simulink model "h2omnix_heading_coop"  (R2022b)
settings: Solver=ode4  StartTime=0.0  StopTime=inf  FixedStep=0.05  RelTol=1e-3
InitFcn:
  | simulacija
undefined symbols (not defined in the file): nu_max, nu_min, pcKd, pcKp, PD_Fil, PD_Filc, PD_Kd, PD_Kdc, PD_Kp, PD_Kpc, vcKi, vcKic, vcKp, vcKpc, vcKt, vcKtc, wn
libraries: MarineRoboticsLib x6, MarineRoboticsLibEx x2, slpidlib x2, matrix_library x2
settings Model: DataDictionary=ros2lib.sldd  Creator=dnad  LastModifiedBy=Zarko Zecevic

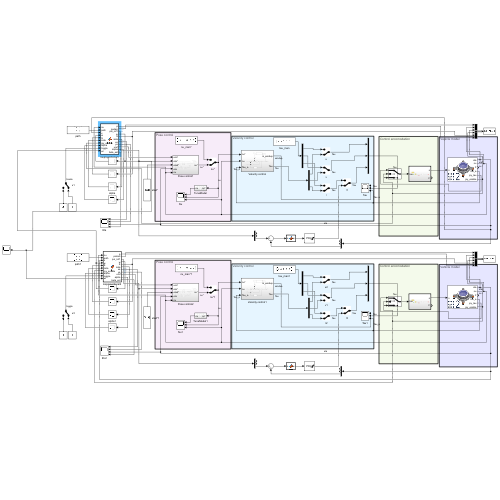
[thumbnail: Simulink's stored preview of the top-level diagram]
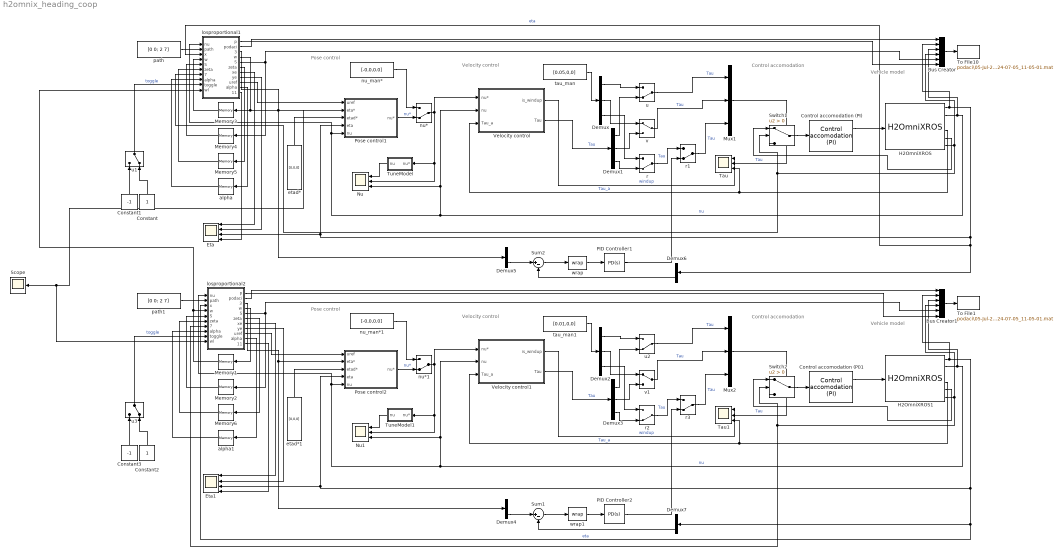
== system h2omnix_heading_coop ==
  note: Control accomodation
  note: Vehicle model
  note: Pose control
  note: Velocity control
  note: Velocity control
  note: Vehicle model
  note: Pose control
  note: Control accomodation
  Bus Creator : BusCreator  Inputs=6
  Bus Creator1 : BusCreator  Inputs=6
  Constant : Constant
  Constant1 : Constant  Value=-1
  Constant2 : Constant
  Constant3 : Constant  Value=-1
  Control accomodation (PI) : MarineRoboticsLibEx/Control accomodation (PI)  SystemSampleTime=-1  VariantActivationTime=update diagram  Latency=0  AutoFrameSizeCalculation=off
  Control accomodation (PI)1 : MarineRoboticsLibEx/Control accomodation (PI)  SystemSampleTime=-1  VariantActivationTime=update diagram  Latency=0  AutoFrameSizeCalculation=off
  Demux{,1..7} (8 alike) : Demux  Outputs=3
  Eta : Scope  NumInputPorts=4
  Eta1 : Scope  NumInputPorts=4
  H2OmniXROS : MarineRoboticsLib/H2OmniXROS  vehicle_name=krk  max_pwm=0.4  pwm_topic=/krk/pwm_out  joy_topic=/krk/joy  odometry_topic=/krk/odometry/filtered
  H2OmniXROS1 : MarineRoboticsLib/H2OmniXROS  vehicle_name=cres  max_pwm=0.4  pwm_topic=/cres/pwm_out  joy_topic=/cres/joy  odometry_topic=/cres/odometry/filtered
  Memory1 : Memory  InitialCondition=1
  Memory2 : Memory  InitialCondition=0.1*eye(3)
  Memory3 : Memory  InitialCondition=1
  Memory4 : Memory  InitialCondition=0.1*eye(3)
  Memory5 : Memory  InitialCondition=[0;0;0]
  Memory6 : Memory  InitialCondition=[0;0;0]
  Mux1 : Mux  Inputs=3
  Mux2 : Mux  Inputs=3
  Nu : Scope  NumInputPorts=3
  Nu1 : Scope  NumInputPorts=3
  PID Controller1 : slpidlib/PID Controller  Controller=PD  Form=Parallel  TimeDomain=Continuous-time  UseExternalTs=off  SampleTime=-1  IntegratorMethod=Forward Euler  FilterMethod=Forward Euler  ControllerParametersSource=internal  P=PD_Kp  I=1  UseKiTs=off  D=PD_Kd  N=PD_Fil  UseFilter=on  TunerSelectOption=Transfer Function Based (PID Tuner App)  InitialConditionSource=internal  InitialConditionForIntegrator=0  InitialConditionForFilter=0  DifferentiatorICPrevScaledInput=0  ExternalReset=none  TrackingMode=off  Kt=1  LimitOutput=on  SatLimitsSource=internal  UpperSaturationLimit=0.8  LowerSaturationLimit=-0.8  LinearizeAsGain=on  AntiWindupMode=none  Kb=1  LimitIntegrator=off  UpperIntegratorSaturationLimit=inf  LowerIntegratorSaturationLimit=-inf  POutMin=[]  POutMax=[]  IOutMin=[]  IOutMax=[]  DOutMin=[]  DOutMax=[]  NOutMin=[]  NOutMax=[]  SumOutMin=[]  SumOutMax=[]  SaturationOutMin=[]  SaturationOutMax=[]  PParamMin=[]  PParamMax=[]  IParamMin=[]  IParamMax=[]  DParamMin=[]  DParamMax=[]  NParamMin=[]  NParamMax=[]  KbParamMin=[]  KbParamMax=[]  KtParamMin=[]  KtParamMax=[]  KbOutMin=[]  KbOutMax=[]  KtOutMin=[]  KtOutMax=[]  IntegratorOutMin=[]  IntegratorOutMax=[]  FilterOutMin=[]  FilterOutMax=[]  SumI1OutMin=[]  SumI1OutMax=[]  SumI2OutMin=[]  SumI2OutMax=[]  SumI3OutMin=[]  SumI3OutMax=[]  SumI4OutMin=[]  SumI4OutMax=[]  SumDOutMin=[]  SumDOutMax=[]  DifferentiatorOutMin=[]  DifferentiatorOutMax=[]  FilterDiffOutCoefMin=[]  FilterDiffOutCoefMax=[]  ReciprocalOutMin=[]  ReciprocalOutMax=[]  SumDenOutMin=[]  SumDenOutMax=[]  SumNumOutMin=[]  SumNumOutMax=[]  DivideOutMin=[]  DivideOutMax=[]  UdiffTsProdOutMin=[]  UdiffTsProdOutMax=[]  NTsProdOutMin=[]  NTsProdOutMax=[]  UintegralTsProdOutMin=[]  UintegralTsProdOutMax=[]  UngainTsProdOutMin=[]  UngainTsProdOutMax=[]  ClampingZeroOutDataTypeStr=Inherit: Inherit via back propagation  ClampingZeroOutMin=[]  ClampingZeroOutMax=[]  FilterDenConstantOutDataTypeStr=Inherit: Inherit via back propagation  FilterDenConstantOutMin=[]  FilterDenConstantOutMax=[]  PCopyOutDataTypeStr=Inherit: Inherit via back propagation  PCopyOutMin=[]  PCopyOutMax=[]  NCopyOutDataTypeStr=Inherit: Inherit via back propagation  NCopyOutMin=[]  NCopyOutMax=[]  IntegratorContinuousStateAttributes=''  IntegratorStateMustResolveToSignalObject=off  IntegratorRTWStateStorageClass=Auto  FilterContinuousStateAttributes=''  FilterStateMustResolveToSignalObject=off  FilterRTWStateStorageClass=Auto  ParallelPVariant=InternalParameters  IdealPVariant=Disabled  IVariant=Disabled  DVariant=InternalParameters  IntegratorVariant=Disabled  SatVariant=Enabled  AWVariant=Disabled  PCopyVariant=Disabled  TRVariant=Disabled  FdbkBlocksVariant=Forward  IdealPFdbkVariant=Disabled  SatFdbkVariant=Disabled  DerivativeFilterVariant=ContFilter  NVariant=InternalParameters  NCopyVariant=Disabled  FilterICVariant=InternalICsFilter  IntegratorICVariant=Disabled  ExternalResetVariant=Disabled  TRSumVariant=Passthrough  SumFdbkVariant=Disabled  SumVariant=Sum_PD  TsampFilterVariant=InternalTs  TsampNgainVariant=Passthrough  TsampIntegralVariant=Disabled_SignalSpec  ExternalSaturationOutDataTypeStr=Inherit: Same as second input
  PID Controller2 : slpidlib/PID Controller  Controller=PD  Form=Parallel  TimeDomain=Continuous-time  UseExternalTs=off  SampleTime=-1  IntegratorMethod=Forward Euler  FilterMethod=Forward Euler  ControllerParametersSource=internal  P=PD_Kpc  I=1  UseKiTs=off  D=PD_Kdc  N=PD_Filc  UseFilter=on  TunerSelectOption=Transfer Function Based (PID Tuner App)  InitialConditionSource=internal  InitialConditionForIntegrator=0  InitialConditionForFilter=0  DifferentiatorICPrevScaledInput=0  ExternalReset=none  TrackingMode=off  Kt=1  LimitOutput=on  SatLimitsSource=internal  UpperSaturationLimit=0.8  LowerSaturationLimit=-0.8  LinearizeAsGain=on  AntiWindupMode=none  Kb=1  LimitIntegrator=off  UpperIntegratorSaturationLimit=inf  LowerIntegratorSaturationLimit=-inf  POutMin=[]  POutMax=[]  IOutMin=[]  IOutMax=[]  DOutMin=[]  DOutMax=[]  NOutMin=[]  NOutMax=[]  SumOutMin=[]  SumOutMax=[]  SaturationOutMin=[]  SaturationOutMax=[]  PParamMin=[]  PParamMax=[]  IParamMin=[]  IParamMax=[]  DParamMin=[]  DParamMax=[]  NParamMin=[]  NParamMax=[]  KbParamMin=[]  KbParamMax=[]  KtParamMin=[]  KtParamMax=[]  KbOutMin=[]  KbOutMax=[]  KtOutMin=[]  KtOutMax=[]  IntegratorOutMin=[]  IntegratorOutMax=[]  FilterOutMin=[]  FilterOutMax=[]  SumI1OutMin=[]  SumI1OutMax=[]  SumI2OutMin=[]  SumI2OutMax=[]  SumI3OutMin=[]  SumI3OutMax=[]  SumI4OutMin=[]  SumI4OutMax=[]  SumDOutMin=[]  SumDOutMax=[]  DifferentiatorOutMin=[]  DifferentiatorOutMax=[]  FilterDiffOutCoefMin=[]  FilterDiffOutCoefMax=[]  ReciprocalOutMin=[]  ReciprocalOutMax=[]  SumDenOutMin=[]  SumDenOutMax=[]  SumNumOutMin=[]  SumNumOutMax=[]  DivideOutMin=[]  DivideOutMax=[]  UdiffTsProdOutMin=[]  UdiffTsProdOutMax=[]  NTsProdOutMin=[]  NTsProdOutMax=[]  UintegralTsProdOutMin=[]  UintegralTsProdOutMax=[]  UngainTsProdOutMin=[]  UngainTsProdOutMax=[]  ClampingZeroOutDataTypeStr=Inherit: Inherit via back propagation  ClampingZeroOutMin=[]  ClampingZeroOutMax=[]  FilterDenConstantOutDataTypeStr=Inherit: Inherit via back propagation  FilterDenConstantOutMin=[]  FilterDenConstantOutMax=[]  PCopyOutDataTypeStr=Inherit: Inherit via back propagation  PCopyOutMin=[]  PCopyOutMax=[]  NCopyOutDataTypeStr=Inherit: Inherit via back propagation  NCopyOutMin=[]  NCopyOutMax=[]  IntegratorContinuousStateAttributes=''  IntegratorStateMustResolveToSignalObject=off  IntegratorRTWStateStorageClass=Auto  FilterContinuousStateAttributes=''  FilterStateMustResolveToSignalObject=off  FilterRTWStateStorageClass=Auto  ParallelPVariant=InternalParameters  IdealPVariant=Disabled  IVariant=Disabled  DVariant=InternalParameters  IntegratorVariant=Disabled  SatVariant=Enabled  AWVariant=Disabled  PCopyVariant=Disabled  TRVariant=Disabled  FdbkBlocksVariant=Forward  IdealPFdbkVariant=Disabled  SatFdbkVariant=Disabled  DerivativeFilterVariant=ContFilter  NVariant=InternalParameters  NCopyVariant=Disabled  FilterICVariant=InternalICsFilter  IntegratorICVariant=Disabled  ExternalResetVariant=Disabled  TRSumVariant=Passthrough  SumFdbkVariant=Disabled  SumVariant=Sum_PD  TsampFilterVariant=InternalTs  TsampNgainVariant=Passthrough  TsampIntegralVariant=Disabled_SignalSpec  ExternalSaturationOutDataTypeStr=Inherit: Same as second input
  Pose control1 : Subsystem
  Pose control2 : Subsystem
  Scope : Scope
  Sum1 : Sum  Inputs=|+-
  Sum2 : Sum  Inputs=|+-
  Switch1 : Switch  Criteria=u2 > Threshold  SaturateOnIntegerOverflow=off  InputSameDT=off
  Switch2 : Switch  Criteria=u2 > Threshold  SaturateOnIntegerOverflow=off  InputSameDT=off
  Tau : Scope  NumInputPorts=3
  Tau1 : Scope  NumInputPorts=3
  To File1 : ToFile  Filename=podaci\05-Jul-2024\cres_2024-07-05_11-05-01.mat  MatrixName=data  SaveFormat=Timeseries
  To File10 : ToFile  Filename=podaci\05-Jul-2024\krk_2024-07-05_11-05-01.mat  MatrixName=data  SaveFormat=Timeseries
  TuneModel : Subsystem
  TuneModel1 : Subsystem
  Velocity control : Subsystem
  Velocity control1 : Subsystem
  alpha : Memory
  alpha1 : Memory
  etad* : Constant  Value=[0,0,0]
  etad*1 : Constant  Value=[0,0,0]
  losproportional1 : MATLAB Function  TreatAsAtomicUnit=on
  losproportional2 : MATLAB Function  TreatAsAtomicUnit=on
  nu* : ManualSwitch  CurrentSetting=0
  nu*1 : ManualSwitch  CurrentSetting=0
  nu_man* : Constant  Value=[-0,0,0.0]
  nu_man*1 : Constant  Value=[-0,0,0.0]
  path : Constant  Value=[0 0; 2 7]
  path1 : Constant  Value=[0 0; 2 7]
  r{,1..3} (4 alike) : ManualSwitch  CurrentSetting=0
  tau_man : Constant  Value=[0.05,0,0]
  tau_man1 : Constant  Value=[0.01,0,0]
  u{,1..3} (4 alike) : ManualSwitch  CurrentSetting=0
  v : ManualSwitch
  v1 : ManualSwitch
  wrap : MarineRoboticsLib/wrap  SystemSampleTime=-1  VariantActivationTime=update diagram  Latency=0  AutoFrameSizeCalculation=off
      settings: LibrarySourceBlock=|
      | simulink/User-Defined
      | Functions/MATLAB Function
  wrap1 : MarineRoboticsLib/wrap  SystemSampleTime=-1  VariantActivationTime=update diagram  Latency=0  AutoFrameSizeCalculation=off
      settings: LibrarySourceBlock=|
      | simulink/User-Defined
      | Functions/MATLAB Function
  wires:
  Switch1/1 -> Control accomodation (PI)/1
  H2OmniXROS/6 -> losproportional1/7(joy_enable), Switch1/2, Bus Creator/4
  losproportional1/7(xe) -> Eta/1
  Velocity control/1(is_windup) -> Tau/1  "windup"
  etad*/1 -> Pose control1/3(etad*)
  Pose control1/1(nu*) -> nu*/2  "nu*"
  Mux1/1 -> Tau/2, Switch1/3  "Tau"
  TuneModel/1(nu) -> Nu/1
  nu_man*/1 -> nu*/1
  H2OmniXROS/1 -> losproportional1/3(x), Demux6/1, Pose control1/4(eta), Eta/3, Bus Creator/2  "eta"
  H2OmniXROS/2 -> Pose control1/5(nu), losproportional1/1(nu), Velocity control/2(nu), Nu/3, Bus Creator/3  "nu"
  H2OmniXROS/4 -> Velocity control/3(Tau_a), Tau/3  "Tau_a"
  nu*/1 -> Nu/2, TuneModel/1(nu*), Velocity control/1(nu*)
  Velocity control/2(Tau) -> Demux1/1  "Tau"
  Demux/1 -> u/1
  Demux1/1 -> u/2
  Demux/2 -> v/1
  Demux1/2 -> v/2
  Demux/3 -> r/1
  Demux1/3 -> r/2
  v/1 -> Mux1/2  "Tau"
  u/1 -> Mux1/1  "Tau"
  tau_man/1 -> Demux/1
  Control accomodation (PI)/1 -> H2OmniXROS/1
  path/1 -> losproportional1/2(path)
  r/1 -> r1/1  "Tau"
  wrap/1 -> PID Controller1/1
  Sum2/1 -> wrap/1
  PID Controller1/1 -> r1/2
  Demux5/3 -> Sum2/1
  Demux6/3 -> Sum2/2
  r1/1 -> Mux1/3  "Tau"
  H2OmniXROS/5 -> Switch1/1
  Memory3/1 -> losproportional1/4("w ")
  losproportional1/5(S) -> Bus Creator/5, Memory4/1
  Memory4/1 -> losproportional1/5("S ")
  losproportional1/6(zeta) -> Memory5/1
  Memory5/1 -> losproportional1/6("zeta ")
  losproportional1/3(psi_ref1) -> Demux5/1, Pose control1/2(eta*)
  losproportional1/9(uref) -> Pose control1/1(uref)
  losproportional1/2(podaci) -> Bus Creator/1
  Bus Creator/1 -> To File10/1
  losproportional1/10(alpha) -> alpha/1
  alpha/1 -> losproportional1/8("alpha ")
  losproportional1/8(ye) -> Eta/2
  losproportional1/11(beta_est) -> Eta/4
  losproportional1/1(p) -> Bus Creator/6
  u1/1 -> losproportional1/9(toggle)  "toggle"
  Constant/1 -> u1/2
  Constant1/1 -> u1/1
  H2OmniXROS1/1 -> losproportional2/3(x), Demux7/1, Pose control2/4(eta), Eta1/3, Bus Creator1/2  "eta"
  Demux3/1 -> u2/2
  nu*1/1 -> Nu1/2, TuneModel1/1(nu*), Velocity control1/1(nu*)
  TuneModel1/1(nu) -> Nu1/1
  nu_man*1/1 -> nu*1/1
  H2OmniXROS1/4 -> Velocity control1/3(Tau_a), Tau1/3  "Tau_a"
  Mux2/1 -> Tau1/2, Switch2/3  "Tau"
  losproportional2/7(xe) -> Eta1/1
  H2OmniXROS1/2 -> Pose control2/5(nu), losproportional2/1(nu), Velocity control1/2(nu), Nu1/3, Bus Creator1/3  "nu"
  losproportional2/6(zeta) -> Memory6/1
  u3/1 -> losproportional2/9(toggle)  "toggle"
  etad*1/1 -> Pose control2/3(etad*)
  Velocity control1/2(Tau) -> Demux3/1  "Tau"
  losproportional2/2(podaci) -> Bus Creator1/1
  Demux7/3 -> Sum1/2
  losproportional2/11(beta_est) -> Eta1/4
  losproportional2/1(p) -> Bus Creator1/6
  Demux2/2 -> v1/1
  losproportional2/4(w) -> Memory1/1
  alpha1/1 -> losproportional2/8("alpha ")
  Demux2/1 -> u2/1
  Bus Creator1/1 -> To File1/1
  Pose control2/1(nu*) -> nu*1/2  "nu*"
  losproportional2/9(uref) -> Pose control2/1(uref)
  Switch2/1 -> Control accomodation (PI)1/1
  H2OmniXROS1/6 -> losproportional2/7(joy_enable), Switch2/2, Bus Creator1/4
  Memory6/1 -> losproportional2/6("zeta ")
  losproportional2/10(alpha) -> alpha1/1
  Memory2/1 -> losproportional2/5("S ")
  losproportional2/5(S) -> Bus Creator1/5, Memory2/1
  H2OmniXROS1/5 -> Switch2/1
  tau_man1/1 -> Demux2/1
  Sum1/1 -> wrap1/1
  Demux3/3 -> r2/2
  wrap1/1 -> PID Controller2/1
  r3/1 -> Mux2/3  "Tau"
  Demux3/2 -> v1/2
  Demux2/3 -> r2/1
  path1/1 -> losproportional2/2(path)
  Velocity control1/1(is_windup) -> Tau1/1  "windup"
  r2/1 -> r3/1  "Tau"
  Demux4/3 -> Sum1/1
  v1/1 -> Mux2/2  "Tau"
  u2/1 -> Mux2/1  "Tau"
  Constant3/1 -> u3/1
  PID Controller2/1 -> r3/2
  losproportional2/8(ye) -> Eta1/2
  Control accomodation (PI)1/1 -> H2OmniXROS1/1
  Constant2/1 -> u3/2
  losproportional2/3(psi_ref1) -> Demux4/1, Pose control2/2(eta*)
  Memory1/1 -> losproportional1/10(wl), losproportional2/4("w ")
  losproportional1/4(w) -> losproportional2/10(wl), Scope/1, Memory3/1

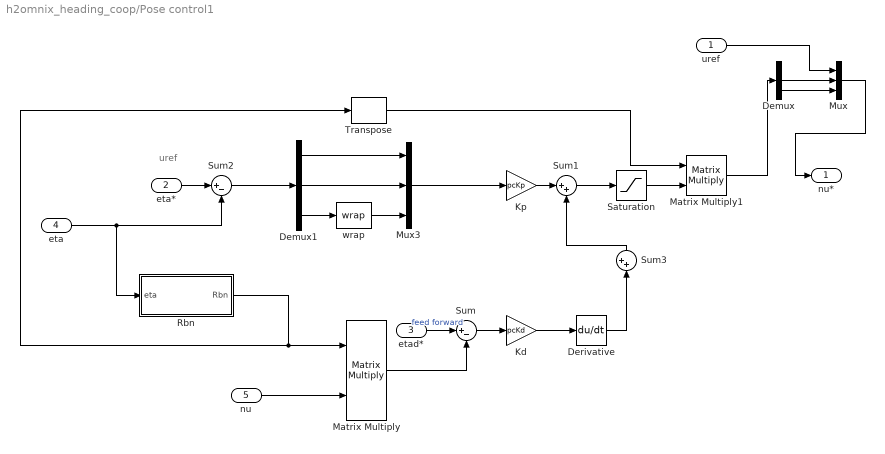
== system h2omnix_heading_coop/Pose control1 ==
  note: uref
  uref : Inport
  eta* : Inport  Port=2
  etad* : Inport  Port=3
  eta : Inport  Port=4
  nu : Inport  Port=5
  Demux : Demux  Outputs=3
  Demux1 : Demux  Outputs=3
  Derivative : Derivative
  Kd : Gain  Gain=pcKd
  Kp : Gain  Gain=pcKp
  Matrix Multiply : Product  Multiplication=Matrix(*)
  Matrix Multiply1 : Product  Multiplication=Matrix(*)
  Mux : Mux  Inputs=3
  Mux3 : Mux  Inputs=3
  Rbn : MATLAB Function  TreatAsAtomicUnit=on
  Saturation : Saturate  UpperLimit=nu_max  LowerLimit=nu_min
  Sum : Sum  Inputs=|+-
  Sum1 : Sum  Inputs=|++
  Sum2 : Sum  Inputs=|+-
  Sum3 : Sum  Inputs=++|
  Transpose : matrix_library/Transpose
  wrap : MarineRoboticsLib/wrap  SystemSampleTime=-1  VariantActivationTime=update diagram  Latency=0  AutoFrameSizeCalculation=off
      settings: LibrarySourceBlock=|
      | simulink/User-Defined
      | Functions/MATLAB Function
  nu* : Outport
  wires:
  Sum/1 -> Kd/1
  eta/1 -> Rbn/1(eta), Sum2/2
  etad*/1 -> Sum/1  "feed forward"
  Kp/1 -> Sum1/1
  eta*/1 -> Sum2/1
  Sum2/1 -> Demux1/1
  Demux1/1 -> Mux3/1
  Demux1/2 -> Mux3/2
  Demux1/3 -> wrap/1
  wrap/1 -> Mux3/3
  Mux3/1 -> Kp/1
  Sum1/1 -> Saturation/1
  Sum3/1 -> Sum1/2
  Kd/1 -> Derivative/1
  Rbn/1(Rbn) -> Matrix Multiply/1, Transpose/1
  Matrix Multiply1/1 -> Demux/1
  Matrix Multiply/1 -> Sum/2
  Saturation/1 -> Matrix Multiply1/2
  Transpose/1 -> Matrix Multiply1/1
  Derivative/1 -> Sum3/2
  nu/1 -> Matrix Multiply/2
  Demux/3 -> Mux/3
  Demux/2 -> Mux/2
  uref/1 -> Mux/1
  Mux/1 -> nu*/1

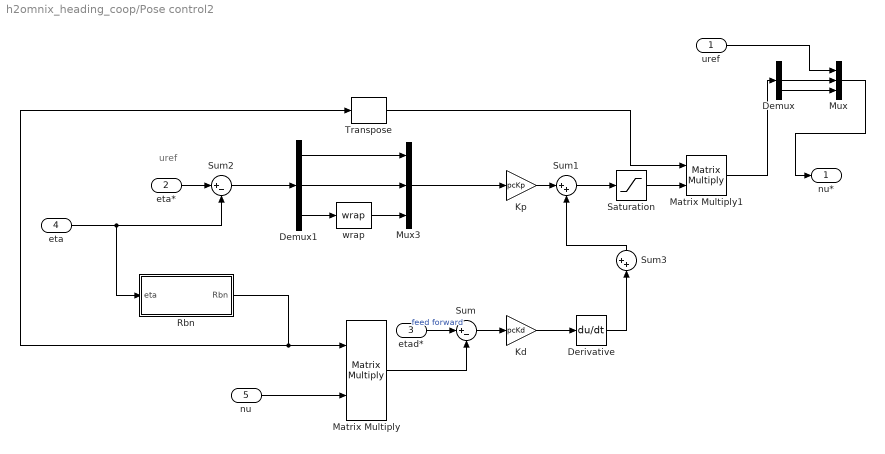
== system h2omnix_heading_coop/Pose control2 ==
  note: uref
  uref : Inport
  eta* : Inport  Port=2
  etad* : Inport  Port=3
  eta : Inport  Port=4
  nu : Inport  Port=5
  Demux : Demux  Outputs=3
  Demux1 : Demux  Outputs=3
  Derivative : Derivative
  Kd : Gain  Gain=pcKd
  Kp : Gain  Gain=pcKp
  Matrix Multiply : Product  Multiplication=Matrix(*)
  Matrix Multiply1 : Product  Multiplication=Matrix(*)
  Mux : Mux  Inputs=3
  Mux3 : Mux  Inputs=3
  Rbn : MATLAB Function  TreatAsAtomicUnit=on
  Saturation : Saturate  UpperLimit=nu_max  LowerLimit=nu_min
  Sum : Sum  Inputs=|+-
  Sum1 : Sum  Inputs=|++
  Sum2 : Sum  Inputs=|+-
  Sum3 : Sum  Inputs=++|
  Transpose : matrix_library/Transpose
  wrap : MarineRoboticsLib/wrap  SystemSampleTime=-1  VariantActivationTime=update diagram  Latency=0  AutoFrameSizeCalculation=off
      settings: LibrarySourceBlock=|
      | simulink/User-Defined
      | Functions/MATLAB Function
  nu* : Outport
  wires:
  Sum/1 -> Kd/1
  eta/1 -> Rbn/1(eta), Sum2/2
  etad*/1 -> Sum/1  "feed forward"
  Kp/1 -> Sum1/1
  eta*/1 -> Sum2/1
  Sum2/1 -> Demux1/1
  Demux1/1 -> Mux3/1
  Demux1/2 -> Mux3/2
  Demux1/3 -> wrap/1
  wrap/1 -> Mux3/3
  Mux3/1 -> Kp/1
  Sum1/1 -> Saturation/1
  Sum3/1 -> Sum1/2
  Kd/1 -> Derivative/1
  Rbn/1(Rbn) -> Matrix Multiply/1, Transpose/1
  Matrix Multiply1/1 -> Demux/1
  Matrix Multiply/1 -> Sum/2
  Saturation/1 -> Matrix Multiply1/2
  Transpose/1 -> Matrix Multiply1/1
  Derivative/1 -> Sum3/2
  nu/1 -> Matrix Multiply/2
  Demux/3 -> Mux/3
  Demux/2 -> Mux/2
  uref/1 -> Mux/1
  Mux/1 -> nu*/1

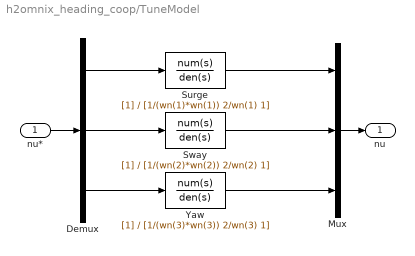
== system h2omnix_heading_coop/TuneModel ==
  nu* : Inport
  Demux : Demux  Outputs=3
  Mux : Mux  Inputs=3
  Surge : TransferFcn  Denominator=[1/(wn(1)*wn(1)) 2/wn(1) 1]
  Sway : TransferFcn  Denominator=[1/(wn(2)*wn(2)) 2/wn(2) 1]
  Yaw : TransferFcn  Denominator=[1/(wn(3)*wn(3)) 2/wn(3) 1]
  nu : Outport
  wires:
  nu*/1 -> Demux/1
  Demux/1 -> Surge/1
  Surge/1 -> Mux/1
  Mux/1 -> nu/1
  Sway/1 -> Mux/2
  Demux/2 -> Sway/1
  Demux/3 -> Yaw/1
  Yaw/1 -> Mux/3

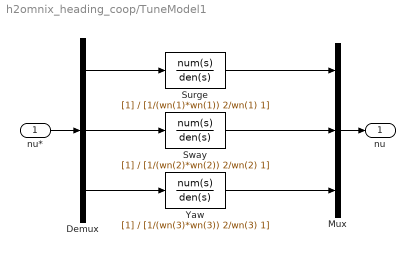
== system h2omnix_heading_coop/TuneModel1 ==
  nu* : Inport
  Demux : Demux  Outputs=3
  Mux : Mux  Inputs=3
  Surge : TransferFcn  Denominator=[1/(wn(1)*wn(1)) 2/wn(1) 1]
  Sway : TransferFcn  Denominator=[1/(wn(2)*wn(2)) 2/wn(2) 1]
  Yaw : TransferFcn  Denominator=[1/(wn(3)*wn(3)) 2/wn(3) 1]
  nu : Outport
  wires:
  nu*/1 -> Demux/1
  Demux/1 -> Surge/1
  Surge/1 -> Mux/1
  Mux/1 -> nu/1
  Sway/1 -> Mux/2
  Demux/2 -> Sway/1
  Demux/3 -> Yaw/1
  Yaw/1 -> Mux/3

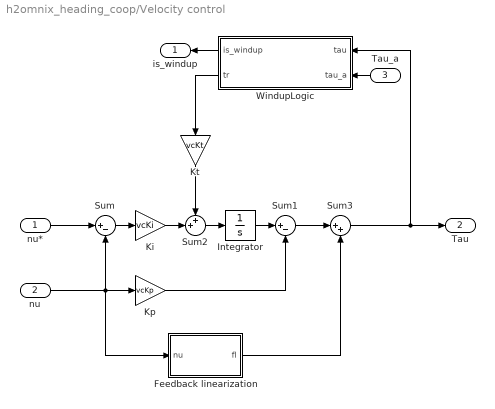
== system h2omnix_heading_coop/Velocity control ==
  nu* : Inport
  nu : Inport  Port=2
  Tau_a : Inport  Port=3
  Feedback linearization : MATLAB Function  TreatAsAtomicUnit=on
  Integrator : Integrator
  Ki : Gain  Gain=vcKi
  Kp : Gain  Gain=vcKp
  Kt : Gain  Gain=vcKt
  Sum : Sum  Inputs=|+-
  Sum1 : Sum  Inputs=|+-
  Sum2 : Sum  Inputs=++|
  Sum3 : Sum  Inputs=|++
  WindupLogic : MATLAB Function  TreatAsAtomicUnit=on
  is_windup : Outport
  Tau : Outport  Port=2
  wires:
  Tau_a/1 -> WindupLogic/2(tau_a)
  nu/1 -> Feedback linearization/1(nu), Kp/1, Sum/2
  Integrator/1 -> Sum1/1
  nu*/1 -> Sum/1
  Sum/1 -> Ki/1
  Sum2/1 -> Integrator/1
  Kp/1 -> Sum1/2
  Ki/1 -> Sum2/2
  WindupLogic/1(is_windup) -> is_windup/1
  WindupLogic/2(tr) -> Kt/1
  Sum1/1 -> Sum3/1
  Sum3/1 -> WindupLogic/1(tau), Tau/1
  Feedback linearization/1(fl) -> Sum3/2
  Kt/1 -> Sum2/1

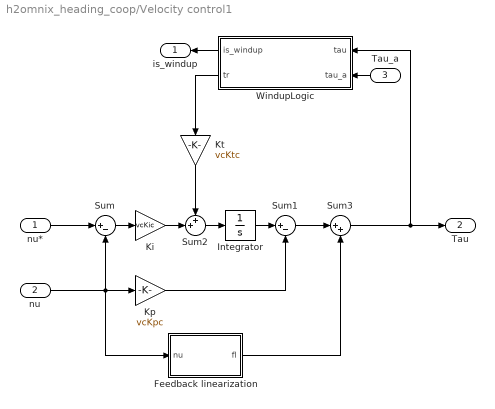
== system h2omnix_heading_coop/Velocity control1 ==
  nu* : Inport
  nu : Inport  Port=2
  Tau_a : Inport  Port=3
  Feedback linearization : MATLAB Function  TreatAsAtomicUnit=on
  Integrator : Integrator
  Ki : Gain  Gain=vcKic
  Kp : Gain  Gain=vcKpc
  Kt : Gain  Gain=vcKtc
  Sum : Sum  Inputs=|+-
  Sum1 : Sum  Inputs=|+-
  Sum2 : Sum  Inputs=++|
  Sum3 : Sum  Inputs=|++
  WindupLogic : MATLAB Function  TreatAsAtomicUnit=on
  is_windup : Outport
  Tau : Outport  Port=2
  wires:
  Tau_a/1 -> WindupLogic/2(tau_a)
  nu/1 -> Feedback linearization/1(nu), Kp/1, Sum/2
  Integrator/1 -> Sum1/1
  nu*/1 -> Sum/1
  Sum/1 -> Ki/1
  Sum2/1 -> Integrator/1
  Kp/1 -> Sum1/2
  Ki/1 -> Sum2/2
  WindupLogic/1(is_windup) -> is_windup/1
  WindupLogic/2(tr) -> Kt/1
  Sum1/1 -> Sum3/1
  Sum3/1 -> WindupLogic/1(tau), Tau/1
  Feedback linearization/1(fl) -> Sum3/2
  Kt/1 -> Sum2/1

== matlab function h2omnix_heading_coop/losproportional2 ==
  data: p output; nu input; podaci output size=[24 1]; path input; x input; psi_ref1 output size=[3 1]; w input size=[1 1]; w output; S input; S output; zeta input; zeta output; xe output size=[1 1]; ye output size=[1 1]; uref output size=[1 1]; joy_enable input; alpha input; alpha output; beta_est output; toggle input; wl input
function [p,podaci,psi_ref1,w,S,zeta,xe,ye,uref,alpha,beta_est] = plos(nu,path,x,w,S,zeta,joy_enable,alpha,toggle,wl)
%%%%%%%%%%%%%%%%%%%%%%%%%%%%%
alg=1; beta_en=1; u0=0.2;
N=5;
kx=0.5;
Rd=0.1*eye(2);Qd=1*diag([0.1 0.1 0.1]);
Dx=0;Dy=-0.8; %% 
%% alg=1 lider
%% beta_en - koristi se beta
%% u0 brzina lidera
Delta=0.3; % lookahead distance
%%%%%%%%%%%%%%%%%%%%%%%%%%%%
if alg==1
    dx=0;dy=0;
else
    dx=Dx;dy=Dy;
end
wizvod=[wl-dy-w]/0.05;
if alg==2 && N==5
    w=wl-dy;
end
[path(1,1),path(1,2),xp_prim,yp_prim,path_rx,path_ry]=generator(w,N,dx,dy,toggle);
%%
beta_est=atan(zeta(3));dt=0.05; 
alpha_prim=0;
ksi=unwrap([alpha atan2(yp_prim,xp_prim)]);
alpha_prim=[ksi(2)-ksi(1)]/dt;
U=sqrt(nu(1)^2+nu(2)^2);
U=nu(1);
alpha=atan2(yp_prim,xp_prim);
%%
ye=-[x(1)-path(1,1)]*sin(alpha)+[x(2)-path(1,2)]*cos(alpha);
xe=[x(1)-path(1,1)]*cos(alpha)+[x(2)-path(1,2)]*sin(alpha);
%%
if(joy_enable==1)
    S=diag([0.01 0.01 0.01]);
    zeta=[xe;ye;0];
%     zeta=[0;0;0];
%     w=1;    
    w=w+0.05*10*xe/sqrt(xp_prim^2+yp_prim^2);
    up=0;
    uref=u0;
    init=1;
    if N==3
        w=2;
    end
else
    if alg==2
        up=u0;
%         w=w+dt*up/sqrt(xp_prim^2+yp_prim^2);
%         w=w-dy;
%         up=wizvod*sqrt(xp_prim^2+yp_prim^2);
        uref=up-0.2*tanh(2.5*xe);
        if uref>0.45
            uref=0.45;
        end
        if uref<-.45
            uref=-0.45;
        end
    elseif alg==1
        up=U*cos(x(3)-alpha)-U*sin(x(3)-alpha)*beta_est+kx*xe;
        w=w+dt*up/sqrt(xp_prim^2+yp_prim^2);
        uref=u0;
    else
        up=U*cos(x(3)-alpha)-U*sin(x(3)-alpha)*beta_est+kx*xe;
        w=w+dt*up/sqrt(xp_prim^2+yp_prim^2);
        uref=u0;
    end
end
psi_ref=wrapToPi(alpha-atan(ye/Delta+beta_est*beta_en));
%% kalaman

Ak=[0 alpha_prim;-alpha_prim 0];
Fi=[-U*sin(x(3)-alpha);U*cos(x(3)-alpha)];
Bk=[U*cos(x(3)-alpha)-up;U*sin(x(3)-alpha)];
Ck=[1 0;0 1]; %% staviti na [0 0;0 1] da bi sve svelo na varijantu samo sa ye
F=[Ak Fi;0 0 0];H=[Ck [0;0]]; G=[Bk;0];
S=S+dt*[-F'*S-S*F+H'*Rd^-1*H-1*Qd*S];
K=S^-1*H'*Rd^-1;
zeta=zeta+dt*(F*zeta+G+K*([xe;ye]-H*zeta));

% psi_ref=0;
psi_ref1=[0;0;psi_ref];
podaci=[alg;xe;ye;psi_ref;w;U;uref;up;Delta;xp_prim;yp_prim;zeta;beta_en;path(1,1);path(1,2);beta_en;alpha_prim;dx;dy;path_rx;path_ry;toggle];
function [x,y,xp_prim,yp_prim,path_rx,path_ry]=generator(w,N,dx,dy,toggle)
switch N
    case 1
        x=(w+dx)*toggle;
        path_rx=w*toggle;
        p=[0 3/7 0];
        y=polyval(p,(w+dx)*toggle)+dy;
        xp_prim=1*toggle;
        yp_prim=2*p(1)*w+p(2);
        path_ry=polyval(p,w*toggle);
    case 2
        x=(w+dx)*toggle;
        path_rx=w*toggle;
        p=[0 3/7 1];
        y=polyval(p,(w+dx)*toggle)+dy;
        xp_prim=1;
        yp_prim=2*p(1)*w+p(2);
        path_ry=polyval(p,w);
    case 3
        x=(w+dx)*toggle;
        path_rx=w*toggle;
        p=[-0.26 1.932 -0.58];
        y=polyval(p,(w+dx))+dy;
        xp_prim=1;
        yp_prim=2*p(1)*w+p(2);
        path_ry=polyval(p,w);
    case 4
        x=(w+dx)*toggle;
        path_rx=w*toggle;
        p=[0.3333 -2.4333 5.2333];
        y=polyval(p,(w+dx))+dy;
        xp_prim=1;
        yp_prim=2*p(1)*w+p(2);
        path_ry=polyval(p,w);
    otherwise
        path_rx=4+2.5*sin(w);
        x=4+2.5*sin(w+dx);
        y=2.1+cos(w+dx);
        xp_prim=2.5*cos(w+dx);
        yp_prim=-sin(w+dx);
        path_ry=2.1+cos(w);
        p=[0 0 0];
end
end
end

== matlab function h2omnix_heading_coop/Velocity control/Feedback linearization ==
  data: nu input; fl output
function fl = feedback_lin(nu)
Betaa = [0, 0, 0]';
fl = Betaa.*abs(nu).*nu;
end

== matlab function h2omnix_heading_coop/Velocity control/WindupLogic ==
  data: tau input; is_windup output; tau_a input; tr output
function [is_windup, tr] = checkWindup(tau, tau_a)
% Consider the tracking within tolerances
tol = 0.01;
is_windup = abs(tau-tau_a)>tol & abs(tau)>0.1;
tr = is_windup.*(tau_a - tau);
end

== matlab function h2omnix_heading_coop/Pose control1/Rbn ==
  data: eta input; Rbn output
function Rbn = RotMatrix(eta)

cp = cos(eta(3));
sp = sin(eta(3));

Rbn = [cp -sp 0;
     sp  cp 0;
      0   0 1];

== matlab function h2omnix_heading_coop/losproportional1 ==
  data: p output; nu input; podaci output size=[24 1]; path input; x input; psi_ref1 output size=[3 1]; w input size=[1 1]; w output; S input; S output; zeta input; zeta output; xe output size=[1 1]; ye output size=[1 1]; uref output size=[1 1]; joy_enable input; alpha input; alpha output; beta_est output; toggle input; wl input
function [p,podaci,psi_ref1,w,S,zeta,xe,ye,uref,alpha,beta_est] = plos(nu,path,x,w,S,zeta,joy_enable,alpha,toggle,wl)
%%%%%%%%%%%%%%%%%%%%%%%%%%%%%
alg=3; beta_en=1; u0=0.2; kx=0.5;
N=5;
Dx=-0.2;Dy=-2; %% 
Rd=0.1*eye(2);Qd=1*diag([0.1 0.1 0.1]);
%% alg=1 lider
%% beta_en - koristi se beta
%% u0 brzina lidera
Delta=1; % lookahead distance
%%%%%%%%%%%%%%%%%%%%%%%%%%%%
if alg==1
    dx=0;dy=0;
else
    dx=Dx;dy=Dy;
end
[path(1,1),path(1,2),xp_prim,yp_prim,path_rx,path_ry]=generator(w,N,dx,dy,toggle);
%%
beta_est=atan(zeta(3));dt=0.05;
alpha_prim=0;
ksi=unwrap([alpha atan2(yp_prim,xp_prim)]);
alpha_prim=[ksi(2)-ksi(1)]/dt;
U=sqrt(nu(1)^2+nu(2)^2);
% U=nu(1);
alpha=atan2(yp_prim,xp_prim);
%%
ye=-[x(1)-path(1,1)]*sin(alpha)+[x(2)-path(1,2)]*cos(alpha);
xe=[x(1)-path(1,1)]*cos(alpha)+[x(2)-path(1,2)]*sin(alpha);
%%
if(joy_enable==1)
    S=diag([0.01 0.01 0.01]);
    zeta=[xe;ye;0];
%     zeta=[0;0;0];
%     w=1;    
    w=w+0.05*10*xe/sqrt(xp_prim^2+yp_prim^2);
    up=0;
    uref=u0;
    init=1;
    if N==3
        w=2;
    end
else
    if alg==2
        up=u0;
        w=w+dt*up/sqrt(xp_prim^2+yp_prim^2);
        uref=up-0.2*tanh(2.5*xe);
        if uref>0.45
            uref=0.45;
        end
        if uref<0
            uref=0.01;
        end
    elseif alg==1
        up=U*cos(x(3)-alpha)-U*sin(x(3)-alpha)*beta_est+kx*xe;
        w=w+dt*up/sqrt(xp_prim^2+yp_prim^2);
        uref=u0;
    else
        up=U*cos(x(3)-alpha)-U*sin(x(3)-alpha)*beta_est+kx*xe;
        w=w+dt*[up/sqrt(xp_prim^2+yp_prim^2)+0.*(wl-w+dy);];
%         uref=u0;
        uref=u0+0.1*tanh(4*(wl-w+dy));
    end
end
psi_ref=wrapToPi(alpha-atan(ye/Delta+beta_est*beta_en));
%% kalaman

Ak=[0 alpha_prim;-alpha_prim 0];
Fi=[-U*sin(x(3)-alpha);U*cos(x(3)-alpha)];
Bk=[U*cos(x(3)-alpha)-up;U*sin(x(3)-alpha)];
Ck=[1 0;0 1]; %% staviti na [0 0;0 1] da bi sve svelo na varijantu samo sa ye
F=[Ak Fi;0 0 0];H=[Ck [0;0]]; G=[Bk;0];
S=S+dt*[-F'*S-S*F+H'*Rd^-1*H-1*Qd*S];
K=S^-1*H'*Rd^-1;
zeta=zeta+dt*(F*zeta+G+K*([xe;ye]-H*zeta));

% psi_ref=-beta_est;
% psi_ref=0;
psi_ref1=[0;0;psi_ref];
podaci=[alg;xe;ye;psi_ref;w;U;uref;up;Delta;xp_prim;yp_prim;zeta;beta_en;path(1,1);path(1,2);beta_en;alpha_prim;dx;dy;path_rx;path_ry;toggle];
function [x,y,xp_prim,yp_prim,path_rx,path_ry]=generator(w,N,dx,dy,toggle)
switch N
    case 1
        x=(w+dx)*toggle;
        path_rx=w*toggle;
        p=[0 3/7 0];
        y=polyval(p,(w+dx)*toggle)+dy;
        xp_prim=1*toggle;
        yp_prim=2*p(1)*w+p(2);
        path_ry=polyval(p,w*toggle);
    case 2
        x=(w+dx)*toggle;
        path_rx=w*toggle;
        p=[0 3/7 1];
        y=polyval(p,(w+dx)*toggle)+dy;
        xp_prim=1;
        yp_prim=2*p(1)*w+p(2);
        path_ry=polyval(p,w);
    case 3
        x=(w+dx)*toggle;
        path_rx=w*toggle;
        p=[-0.26 1.932 -0.58];
        y=polyval(p,(w+dx))+dy;
        xp_prim=1;
        yp_prim=2*p(1)*w+p(2);
        path_ry=polyval(p,w);
    case 4
        x=(w+dx)*toggle;
        path_rx=w*toggle;
        p=[0.3333 -2.4333 5.2333];
        y=polyval(p,(w+dx))+dy;
        xp_prim=1;
        yp_prim=2*p(1)*w+p(2);
        path_ry=polyval(p,w);
    otherwise
        path_rx=4+2.5*sin(w);
        x=4+2.5*sin(w+dx);
        y=2.1+cos(w+dx);
        xp_prim=2.5*cos(w+dx);
        yp_prim=-sin(w+dx);
        path_ry=2.1+cos(w);
        p=[0 0 0];
end
end
end

== matlab function h2omnix_heading_coop/Pose control2/Rbn ==
  data: eta input; Rbn output
function Rbn = RotMatrix(eta)

cp = cos(eta(3));
sp = sin(eta(3));

Rbn = [cp -sp 0;
     sp  cp 0;
      0   0 1];

== matlab function h2omnix_heading_coop/Velocity control1/Feedback linearization ==
  data: nu input; fl output
function fl = feedback_lin(nu)
Betaa = [0, 0, 0]';
fl = Betaa.*abs(nu).*nu;
end

== matlab function h2omnix_heading_coop/Velocity control1/WindupLogic ==
  data: tau input; is_windup output; tau_a input; tr output
function [is_windup, tr] = checkWindup(tau, tau_a)
% Consider the tracking within tolerances
tol = 0.01;
is_windup = abs(tau-tau_a)>tol & abs(tau)>0.1;
tr = is_windup.*(tau_a - tau);
end
